simulink model "adcs_v11_log"  (Simulink 7.4)
settings: Solver=ode4  StartTime=0.0  StopTime=80000  FixedStep=s_SIM_STEP_SIZE  RelTol=1e-3
values from neighbouring files (symbols this model uses):
  A = ((T_SIDE + .29)*1e-3)^2    [constants_v13.m]    (also in constants_v15.m; constants_v15_Pow.m; constants_v15_Pow_ss_error.m; constants_v16_integral_kartavya.m)
  Ca_Solar_Drag = 1.4    [constants_v13.m]    (also in constants_v15.m; constants_v15_Pow.m; constants_v15_Pow_ss_error.m; constants_v16_integral_kartavya.m)
  Cd = 2.2    [constants_v13.m]    (also in constants_v15.m; constants_v15_Pow.m; constants_v15_Pow_ss_error.m; constants_v16_integral_kartavya.m)
  check_time = 60000    [constants_v13.m]    (also in constants_v15.m = 10000; constants_v15_Pow.m = 10000; constants_v15_Pow_ss_error.m = 10000; constants_v16_integral_kartavya.m = 10000)
  equinox = datenum('21-Mar-2010 12:0:0')    [constants_v13.m]    (also in constants_v15.m; constants_v15_Pow.m; constants_v15_Pow_ss_error.m; constants_v16_integral_kartavya.m)
  err_SGP = 0    [constants_v16_integral_kartavya.m]    (also in constants_v16_integral_light_sun_sgp_igrf_power_13Dec2011.m)
  I_MAX = 0.5    [constants_v13.m]    (also in constants_v15.m; constants_v15_Pow.m; constants_v15_Pow_ss_error.m; constants_v16_integral_kartavya.m)
  I_TORQUER = 3.6 / 7.31    (= 0.492476060192)    [constants_v13.m]    (also in constants_v15.m; constants_v15_Pow.m; constants_v15_Pow_ss_error.m; constants_v16_integral_kartavya.m)
  Kd = 2* m_INERTIA / (s_numOrbits * T_ORBIT )    [constants_v13.m]    (also in constants_v15.m = m_INERTIA * (2 + delta)* zeta * w; constants_v15_Pow.m = m_INERTIA * (2 + delta)* zeta * w; constants_v15_Pow_ss_error.m = m_INERTIA * (2 + delta)* zeta * w; constants_v16_integral_kartavya.m = m_INERTIA * (2 + delta)* zeta * w)
  Kdetumb = K_det*eye(3)    [constants_v13.m]    (also in constants_v15.m; constants_v15_Pow.m; constants_v15_Pow_ss_error.m; constants_v16_integral_kartavya.m)
  Kp = m_INERTIA / (s_numOrbits * T_ORBIT * zeta)^2    [constants_v13.m]    (also in constants_v15.m = m_INERTIA * (w*w + 2*delta*zeta^2*w^2); constants_v15_Pow.m = m_INERTIA * (w*w + 2*delta*zeta^2*w^2); constants_v15_Pow_ss_error.m = m_INERTIA * (w*w + 2*delta*zeta^2*w^2); constants_v16_integral_kartavya.m = m_INERTIA * (w*w + 2*delta*zeta^2*w^2))
  m_INERTIA = [Ixx Ixy Ixz; Ixy Iyy Iyz; Ixz Iyz Izz]    [constants_v13.m]    (also in constants_v15.m; constants_v15_Pow.m = 1*[Ixx Ixy Ixz; Ixy Iyy Iyz; Ixz Iyz Izz]; constants_v15_Pow_ss_error.m = 1*[Ixx Ixy Ixz; Ixy Iyy Iyz; Ixz Iyz Izz]; constants_v16_integral_kartavya.m)
  mu = 6.673e-11*5.9742e24    (= 398658366000000)    [constants_v13.m]    (also in constants_v15.m; constants_v15_Pow.m; constants_v15_Pow_ss_error.m; constants_v16_integral_kartavya.m)
  N = 40    [constants_v13.m]    (also in constants_v15.m; constants_v15_Pow.m; constants_v15_Pow_ss_error.m; constants_v16_integral_kartavya.m)
  P_momentum_flux_from_the_sun = 4.4e-6    (= 4.4e-06)    [constants_v13.m]    (also in constants_v15.m; constants_v15_Pow.m; constants_v15_Pow_ss_error.m; constants_v16_integral_kartavya.m)
  q_BI0 = euler2qBI(roll0,pitch0,yaw0)    [constants_v13.m]    (also in constants_v15.m; constants_v15_Pow.m; constants_v15_Pow_ss_error.m; constants_v16_integral_kartavya.m)
  s_AU = 159597870610    [constants_v16_integral_kartavya.m]    (also in constants_v16_integral_light_sun_sgp_igrf_power_13Dec2011.m; light_calc.m)
  s_DOY = sime(2)*30 - 30 + sime(3)    [constants_v16_integral_kartavya.m]    (also in constants_v16_integral_light_sun_sgp_igrf_power_13Dec2011.m; precalcs.m)
  s_FRAME_SIZE = 2    [constants_v13.m]    (also in constants_v15.m; constants_v15_Pow.m; constants_v15_Pow_ss_error.m; constants_v16_integral_kartavya.m)
  s_m_MAX = 0.95    [constants_v13.m]    (also in constants_v15.m; constants_v15_Pow.m; constants_v15_Pow_ss_error.m; constants_v16_integral_kartavya.m)
  s_MAG_B = 2.5e-5    (= 2.5e-05)    [constants_v13.m]    (also in constants_v15.m; constants_v15_Pow.m; constants_v15_Pow_ss_error.m; constants_v16_integral_kartavya.m)
  s_MAGMETER_WEIGHT = .9    (= 0.9)    [constants_v13.m]    (also in constants_v15.m; constants_v15_Pow.m; constants_v15_Pow_ss_error.m; constants_v16_integral_kartavya.m)
  s_Rearth = 6378164    [constants_v16_integral_kartavya.m]    (also in constants_v16_integral_light_sun_sgp_igrf_power_13Dec2011.m; light_calc.m)
  s_Rsun = 695500000    [constants_v16_integral_kartavya.m]    (also in constants_v16_integral_light_sun_sgp_igrf_power_13Dec2011.m; light_calc.m)
  s_SEC = sime(4)*3600 + sime(5)*60 + sime(6)    [constants_v16_integral_kartavya.m]    (also in constants_v16_integral_light_sun_sgp_igrf_power_13Dec2011.m; precalcs.m)
  s_SIM_STEP_SIZE = 0.1    [constants_v13.m]    (also in constants_v15.m; constants_v15_Pow.m; constants_v15_Pow_ss_error.m; constants_v16_integral_kartavya.m)
  s_SS_ADC_gain = 5    [constants_v13.m]    (also in constants_v15.m; constants_v15_Pow.m; constants_v15_Pow_ss_error.m; constants_v16_integral_kartavya.m)
  s_SS_ADC_res = 2^12 - 1    (= 4095)    [constants_v13.m]    (also in constants_v15.m; constants_v15_Pow.m; constants_v15_Pow_ss_error.m; constants_v16_integral_kartavya.m)
  s_SS_MAX_ANGLE = 85    [constants_v13.m]    (also in constants_v15.m; constants_v15_Pow.m; constants_v15_Pow_ss_error.m; constants_v16_integral_kartavya.m)
  s_W_SAT = sqrt(mu/R_e^3)    [constants_v13.m]    (also in constants_v15.m; constants_v15_Pow.m; constants_v15_Pow_ss_error.m; constants_v16_integral_kartavya.m)
  s_x_MAGMETER_BIAS = 50e-9    (= 5e-08)    [constants_v13.m]    (also in constants_v15.m; constants_v15_Pow.m; constants_v15_Pow_ss_error.m; constants_v16_integral_kartavya.m)
  s_YEAR = sime(1) + (sime(2)*30 - 30 + sime(3))/365    [constants_v16_integral_kartavya.m]    (also in constants_v16_integral_light_sun_sgp_igrf_power_13Dec2011.m; precalcs.m)
  side = 0.26    [constants_v13.m]    (also in constants_v15.m; constants_v15_Pow.m; constants_v15_Pow_ss_error.m; constants_v16_integral_kartavya.m)
  Snum = 6    [constants_v13.m]    (also in constants_v15.m; constants_v15_Pow.m; constants_v15_Pow_ss_error.m; constants_v16_integral_kartavya.m)
  stperut = 1.00273790935    [constants_v16_integral_kartavya.m]    (also in constants_v16_integral_light_sun_sgp_igrf_power_13Dec2011.m; precalcs.m)
  t_reset = 600    [constants_v16_integral_kartavya.m]    (also in constants_v16_integral_light_sun_sgp_igrf_power_13Dec2011.m; precalcs.m)
  TLE_epoch = datenum('18-Oct-2010 10:30:0')    [constants_v16_integral_kartavya.m]    (also in constants_v16_integral_light_sun_sgp_igrf_power_13Dec2011.m; precalcs.m)
  today = datenum('18-Oct-2010 10:30:0')    [constants_v13.m]    (also in constants_v15.m; constants_v15_Pow.m; constants_v15_Pow_ss_error.m; constants_v16_integral_kartavya.m)
  tol_w = 4e-3    (= 0.004)    [constants_v13.m]    (also in constants_v15.m; constants_v15_Pow.m; constants_v15_Pow_ss_error.m; constants_v16_integral_kartavya.m)
  Ts_display = 6    [constants_v13.m]    (also in constants_v15.m; constants_v15_Pow.m; constants_v15_Pow_ss_error.m; constants_v16_integral_kartavya.m)
  v_COM_to_COP_b = [.2; 1.75; .2]*1e-2    [constants_v13.m]    (also in constants_v15.m; constants_v15_Pow.m; constants_v15_Pow_ss_error.m; constants_v16_integral_kartavya.m)
  v_S1 = [1 0 0]    [constants_v13.m]    (also in constants_v15.m; constants_v15_Pow.m; constants_v15_Pow_ss_error.m; constants_v16_integral_kartavya.m)
  v_S2 = [-1 0 0]    [constants_v13.m]    (also in constants_v15.m; constants_v15_Pow.m; constants_v15_Pow_ss_error.m; constants_v16_integral_kartavya.m)
  v_S3 = [0 1 0]    [constants_v13.m]    (also in constants_v15.m; constants_v15_Pow.m; constants_v15_Pow_ss_error.m; constants_v16_integral_kartavya.m)
  v_S4 = [0 -1 0]    [constants_v13.m]    (also in constants_v15.m; constants_v15_Pow.m; constants_v15_Pow_ss_error.m; constants_v16_integral_kartavya.m)
  v_S5 = [0 0 1]    [constants_v13.m]    (also in constants_v15.m; constants_v15_Pow.m; constants_v15_Pow_ss_error.m; constants_v16_integral_kartavya.m)
  v_S6 = [0 0 -1]    [constants_v13.m]    (also in constants_v15.m; constants_v15_Pow.m; constants_v15_Pow_ss_error.m; constants_v16_integral_kartavya.m)
  v_x_MOUNTING_THETA_ZYX_BODY_TORQUER = [1; 1; 1]* pi/180    [constants_v13.m]    (also in constants_v15.m; constants_v15_Pow.m; constants_v15_Pow_ss_error.m; constants_v16_integral_kartavya.m)
  W_EARTH_ROT = 2*pi/86400    (= 7.27220521664e-05)    [constants_v16_integral_kartavya.m]    (also in constants_v16_integral_light_sun_sgp_igrf_power_13Dec2011.m; precalcs.m)
  wx0 = 2*pi/180    (= 0.0349065850399)    [constants_v13.m]    (also in constants_v15.m = 0.00174532925199; constants_v15_Pow.m = 1.74532925199e-05; constants_v15_Pow_ss_error.m = 2.01533262693e-05; constants_v16_integral_kartavya.m = 0.0174532925199)
  wy0 = 1*pi/180    (= 0.0174532925199)    [constants_v13.m]    (also in constants_v15.m = 0.00174532925199; constants_v15_Pow.m = 1.74532925199e-05; constants_v15_Pow_ss_error.m = 2.01533262693e-05; constants_v16_integral_kartavya.m = 0)
  wz0 = -2*pi/180    (= -0.0349065850399)    [constants_v13.m]    (also in constants_v15.m = 0.00174532925199; constants_v15_Pow.m = 1.74532925199e-05; constants_v15_Pow_ss_error.m = 2.01533262693e-05; constants_v16_integral_kartavya.m = -0.00872664625997)
undefined symbols (not defined in the file or in its folder): Earth, s_omega_MAX, s_YEAR_ONLY, tol_pitch, tol_roll, tol_yaw, v_S10, v_S11, v_S12, v_S7, v_S8, v_S9, v_Si0, WGS84
libraries: commnoisgen2 x15, aerolibutil x7, aerolibtransform2 x5, dspsigops x5, powerlib_extras x3, aerolibgravity2 x2, aerolibatmos2 x1, dspmtrx3 x1, simulink x1
(part 1 of 3)
settings Model: Creator=Jaideep  LastModifiedBy=Jaideep  SimulationMode=rapid-accelerator  ExtModeTrigDuration=100
settings SolverCC: AutoInsertRateTranBlk=on
settings DataIOCC: SaveFinalState=on  SaveOutput=off  SaveState=on  StateSaveName=tmp_raccel_xout
settings OptimizationCC: EfficientMapNaN2IntZero=off
settings HardwareCC: TargetEndianess=LittleEndian  TargetHWDeviceType=MATLAB Host  ProdEqTarget=off
settings RTWCC: SystemTargetFile=raccel.tlc  TemplateMakefile=raccel_default_tmf  RTWVerbose=off  ProcessScript=raccel_make_rtw_hook
settings CodeAppCC: GenerateComments=off  MaxIdLength=128  SimulinkBlockComments=off
settings RaccelTargetCC: TargetFunctionLibrary=ANSI_C  ERTMultiwordTypeDef=System defined  ERTMultiwordLength=256  IsPILTarget=off  ParMdlRefBuildCompliant=off  GeneratePreprocessorConditionals=Disable all  ERTFirstTimeCompliant=off  MultiInstanceERTCode=off  EnableShiftOperators=on  PortableWordSizes=off  ExtModeMexArgs='', 0, 7081  RTWCAPISignals=off  RTWCAPIParams=off

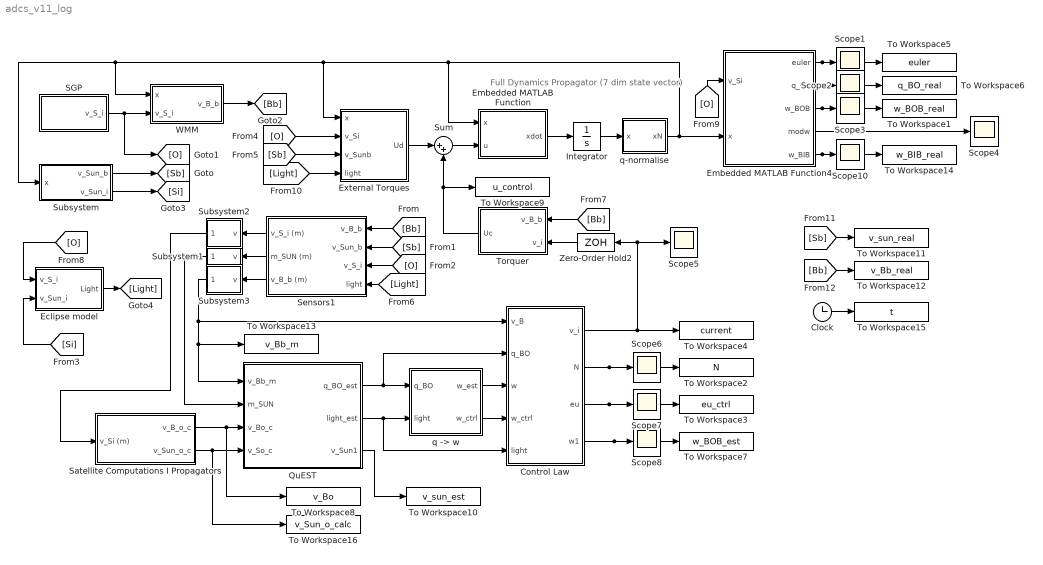
== system adcs_v11_log ==
  note: Full Dynamics Propagator
      |  (7 dim state vector)
  Clock : Clock
      settings: Decimation=10
  Control Law : Subsystem
  Eclipse model : Subsystem
  Embedded MATLAB Function : Stateflow chart
  Embedded MATLAB Function4 : Stateflow chart
  External Torques : Subsystem
  Integrator : Integrator  InitialCondition=[q_BI0; wx0; wy0; wz0]
  QuEST : Stateflow chart
  "SGP " : Subsystem
  Satellite Computations I Propagators : Subsystem
  Scope{1..8,10} (9 alike) : Scope
      Scope1 settings: TimeRange=80000  YMin=-200  YMax=200  SampleInput=on  SampleTime=5
      Scope10 settings: YMin=0.004  YMax=0.0075  SaveName=ScopeData23  SampleInput=on  SampleTime=5
      Scope2 settings: YMin=-10  YMax=10  SaveName=ScopeData7  SampleInput=on  SampleTime=5
      Scope3 settings: YMin=-10  YMax=10  SaveName=ScopeData14  SampleInput=on  SampleTime=5
      Scope4 settings: YMin=0.004  YMax=0.0075  SaveName=ScopeData21  SampleInput=on  SampleTime=5
      Scope5 settings: YMin=-0.045  YMax=0.04  SaveName=ScopeData11  SampleInput=on  SampleTime=5
      Scope6 settings: YMin=-1  YMax=1  SaveName=ScopeData15  SampleInput=on  SampleTime=5
      Scope7 settings: YMin=-10  YMax=10  SaveName=ScopeData16  SampleInput=on  SampleTime=5
      Scope8 settings: YMin=-10  YMax=10  SaveName=ScopeData20  SampleInput=on  SampleTime=5
  Sensors1 : Subsystem
  Subsystem : Subsystem
  Subsystem1 : Subsystem
  Subsystem2 : Subsystem
  Subsystem3 : Subsystem
  Sum : Sum  Inputs=|++  OutDataType=sfix(16)  OutScaling=2^0
  To Workspace1 : ToWorkspace  VariableName=w_BOB_real  SampleTime=Ts_display  SaveFormat=Array
  To Workspace10 : ToWorkspace  VariableName=v_sun_est  SampleTime=Ts_display  SaveFormat=Array
  To Workspace11 : ToWorkspace  VariableName=v_sun_real  SampleTime=Ts_display  SaveFormat=Array
  To Workspace12 : ToWorkspace  VariableName=v_Bb_real  SampleTime=Ts_display  SaveFormat=Array
  To Workspace13 : ToWorkspace  VariableName=v_Bb_m  SampleTime=Ts_display  SaveFormat=Array
  To Workspace14 : ToWorkspace  VariableName=w_BIB_real  SampleTime=Ts_display  SaveFormat=Array
  To Workspace15 : ToWorkspace  VariableName=t  SampleTime=Ts_display  SaveFormat=Array
  To Workspace16 : ToWorkspace  VariableName=v_Sun_o_calc  SampleTime=Ts_display  SaveFormat=Array
  To Workspace2 : ToWorkspace  VariableName=N  SampleTime=Ts_display  SaveFormat=Array
  To Workspace3 : ToWorkspace  VariableName=eu_ctrl  SampleTime=Ts_display  SaveFormat=Array
  To Workspace4 : ToWorkspace  VariableName=current  SampleTime=Ts_display  SaveFormat=Array
  To Workspace5 : ToWorkspace  VariableName=euler  SampleTime=Ts_display  SaveFormat=Array
  To Workspace6 : ToWorkspace  VariableName=q_BO_real  SampleTime=Ts_display  SaveFormat=Array
  To Workspace7 : ToWorkspace  VariableName=w_BOB_est  SampleTime=Ts_display  SaveFormat=Array
  To Workspace8 : ToWorkspace  VariableName=v_Bo  SampleTime=Ts_display  SaveFormat=Array
  To Workspace9 : ToWorkspace  VariableName=u_control  SampleTime=Ts_display  SaveFormat=Array
  Torquer : Subsystem
  WMM : Subsystem
  Zero-Order Hold2 : ZeroOrderHold  SampleTime=s_FRAME_SIZE
  "q -> w" : Subsystem
  q-normalise : Stateflow chart
  wires:
  Embedded MATLAB Function/1(xdot) -> Integrator/1
  Integrator/1 -> q-normalise/1(x)
  "SGP "/1(v_S_i) -> WMM/2(v_S_i), [O]
  q-normalise/1(xN) -> Subsystem/1(x), WMM/1(x), External Torques/1(x), Embedded MATLAB Function/1(x), Embedded MATLAB Function4/2(x)
  Sum/1 -> Embedded MATLAB Function/2(u)
  WMM/1(v_B_b) -> [Bb]
  Subsystem/1(v_Sun_b) -> [Sb]
  [Bb] -> Sensors1/1(v_B_b)
  [Sb] -> Sensors1/2(v_Sun_b)
  Subsystem/2(v_Sun_i) -> [Si]
  [O] -> External Torques/2(v_Si)
  [Sb] -> External Torques/3(v_Sunb)
  [Bb] -> Torquer/1(v_B_b)
  [O] -> Sensors1/3(v_S_i)
  [Light] -> Sensors1/4(light)
  Sensors1/1(v_S_i (m)) -> Subsystem2/1(v)
  [Si] -> Eclipse model/2(v_Sun_i)
  [O] -> Eclipse model/1(v_S_i)
  Sensors1/2(m_SUN (m)) -> Subsystem1/1(v)
  Sensors1/3(v_B_b (m)) -> Subsystem3/1(v)
  Zero-Order Hold2/1 -> Torquer/2(v_i)
  External Torques/1(Ud) -> Sum/1
  Torquer/1(Uc) -> Sum/2, To Workspace9/1
  Subsystem2/1(v(H)) -> Satellite Computations I Propagators/1(v_Si (m))
  Subsystem1/1(v(H)) -> QuEST/2(m_SUN)
  Subsystem3/1(v(H)) -> Control Law/1(v_B), QuEST/1(v_Bb_m), To Workspace13/1
  Satellite Computations I Propagators/1(v_B_o_c) -> QuEST/3(v_Bo_c), To Workspace8/1
  Satellite Computations I Propagators/2(v_Sun_o_c) -> QuEST/4(v_So_c), To Workspace16/1
  QuEST/1(q_BO_est) -> Control Law/2(q_BO), "q -> w"/1(q_BO)
  QuEST/2(light_est) -> "q -> w"/2(light), Control Law/5(light)
  Control Law/1(v_i) -> To Workspace4/1, Zero-Order Hold2/1, Scope5/1
  Embedded MATLAB Function4/2(q_BO) -> Scope2/1, To Workspace6/1
  Embedded MATLAB Function4/1(euler) -> Scope1/1, To Workspace5/1
  [O] -> Embedded MATLAB Function4/1(v_Si)
  Control Law/2(N) -> Scope6/1, To Workspace2/1
  Eclipse model/1(Light) -> [Light]
  Control Law/3(eu) -> Scope7/1, To Workspace3/1
  Embedded MATLAB Function4/3(w_BOB) -> Scope3/1, To Workspace1/1
  Embedded MATLAB Function4/4(modw) -> Scope4/1
  Control Law/4(w1) -> Scope8/1, To Workspace7/1
  "q -> w"/1(w_est) -> Control Law/3(w)
  [Light] -> External Torques/4(light)
  "q -> w"/2(w_ctrl) -> Control Law/4(w_ctrl)
  QuEST/3(v_Sun1) -> To Workspace10/1
  [Sb] -> To Workspace11/1
  [Bb] -> To Workspace12/1
  Embedded MATLAB Function4/5(w_BIB) -> Scope10/1, To Workspace14/1
  Clock/1 -> To Workspace15/1

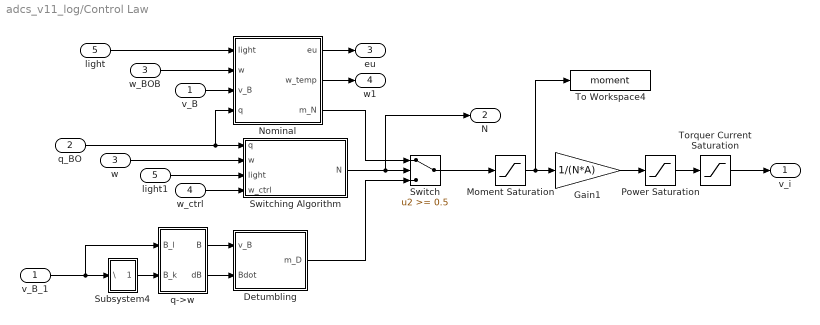
== system adcs_v11_log/Control Law ==
  v_B : Inport  OutDataType=sfix(16)  OutScaling=2^0
  q_BO : Inport  Port=2  OutDataType=sfix(16)  OutScaling=2^0
  w : Inport  Port=3  OutDataType=sfix(16)  OutScaling=2^0
  w_ctrl : Inport  Port=4  OutDataType=sfix(16)  OutScaling=2^0
  light : Inport  Port=5  OutDataType=sfix(16)  OutScaling=2^0
  Detumbling : Stateflow chart
  Gain1 : Gain  Gain=1/(N*A)  ParameterDataType=sfix(16)  ParameterScaling=2^0  OutDataType=sfix(16)  OutScaling=2^0
  Moment Saturation : Saturate  UpperLimit=s_m_MAX  LowerLimit=-s_m_MAX  OutDataType=sfix(16)  OutScaling=2^0
  Nominal : Stateflow chart
  Power Saturation : Saturate  UpperLimit=I_MAX  LowerLimit=-I_MAX  OutDataType=sfix(16)  OutScaling=2^0
  Subsystem4 : Subsystem
  Switch : Switch  Threshold=0.5  OutDataType=sfix(16)  OutScaling=2^0
  Switching Algorithm : Subsystem
  To Workspace4 : ToWorkspace  VariableName=moment  SampleTime=Ts_display  SaveFormat=Array
  Torquer Current Saturation : Saturate  UpperLimit=I_TORQUER  LowerLimit=-I_TORQUER  OutDataType=sfix(16)  OutScaling=2^0
  light1 : InportShadow  Port=5  OutDataType=sfix(16)  OutScaling=2^0  LatchByCopyingInsideSignal=off
  q->w : Stateflow chart
  v_B_1 : InportShadow  Port=1  OutDataType=sfix(16)  OutScaling=2^0  LatchByCopyingInsideSignal=off
  w_BOB : InportShadow  Port=3  OutDataType=sfix(16)  OutScaling=2^0  LatchByCopyingInsideSignal=off
  v_i : Outport  OutDataType=sfix(16)  OutScaling=2^0
  N : Outport  Port=2  OutDataType=sfix(16)  OutScaling=2^0
  eu : Outport  Port=3  OutDataType=sfix(16)  OutScaling=2^0
  w1 : Outport  Port=4  OutDataType=sfix(16)  OutScaling=2^0
  wires:
  q->w/1(B) -> Detumbling/1(v_B)
  Subsystem4/1(=>\) -> q->w/2(B_k)
  q_BO/1 -> Nominal/4(q), Switching Algorithm/1(q)
  light/1 -> Nominal/1(light)
  Gain1/1 -> Power Saturation/1
  Torquer Current Saturation/1 -> v_i/1
  Moment Saturation/1 -> Gain1/1, To Workspace4/1
  Power Saturation/1 -> Torquer Current Saturation/1
  Switch/1 -> Moment Saturation/1
  Detumbling/1(m_D) -> Switch/3
  Switching Algorithm/1(N) -> N/1, Switch/2
  Nominal/3(m_N) -> Switch/1
  w/1 -> Switching Algorithm/2(w)
  v_B_1/1 -> q->w/1(B_l), Subsystem4/1(\)
  q->w/2(dB) -> Detumbling/2(Bdot)
  v_B/1 -> Nominal/3(v_B)
  light1/1 -> Switching Algorithm/3(light)
  w_BOB/1 -> Nominal/2(w)
  Nominal/1(eu) -> eu/1
  Nominal/2(w_temp) -> w1/1
  w_ctrl/1 -> Switching Algorithm/4(w_ctrl)

== system adcs_v11_log/Eclipse model ==
  v_S_i : Inport  OutDataType=sfix(16)  OutScaling=2^0
  v_Sun_i : Inport  Port=2  OutDataType=sfix(16)  OutScaling=2^0
  Constant : Constant  Value=s_AU  OutDataType=sfix(16)  OutScaling=2^0
  Constant1 : Constant  Value=s_Rearth  OutDataType=sfix(16)  OutScaling=2^0
  Constant2 : Constant  Value=s_Rsun  OutDataType=sfix(16)  OutScaling=2^0
  Eclipse Model : Stateflow chart
  Scope{1..4} (4 alike) : Scope
      Scope1 settings: TimeRange=80000  YMin=-6.5  YMax=1  SaveName=ScopeData3  SampleInput=on  SampleTime=5
      Scope2 settings: TimeRange=80000  YMin=-6.5  YMax=1  SaveName=ScopeData4  SampleInput=on  SampleTime=5
      Scope3 settings: TimeRange=80000  YMin=-6.5  YMax=1  SaveName=ScopeData5  SampleInput=on  SampleTime=5
      Scope4 settings: TimeRange=80000  YMin=-6.5  YMax=1  SaveName=ScopeData6  SampleInput=on  SampleTime=5
  Light : Outport  OutDataType=sfix(16)  OutScaling=2^0
  wires:
  Constant/1 -> Eclipse Model/1(s_AU)
  Constant1/1 -> Eclipse Model/2(s_Rearth)
  Constant2/1 -> Eclipse Model/3(s_Rsun)
  Eclipse Model/1(flag) -> Light/1
  v_S_i/1 -> Eclipse Model/4(v_S_i)
  v_Sun_i/1 -> Eclipse Model/5(v_Sun_i)
  Eclipse Model/2(alpha) -> Scope1/1
  Eclipse Model/3(beta) -> Scope2/1
  Eclipse Model/4(parameter_umbra) -> Scope3/1
  Eclipse Model/5(parameter_penumbra) -> Scope4/1

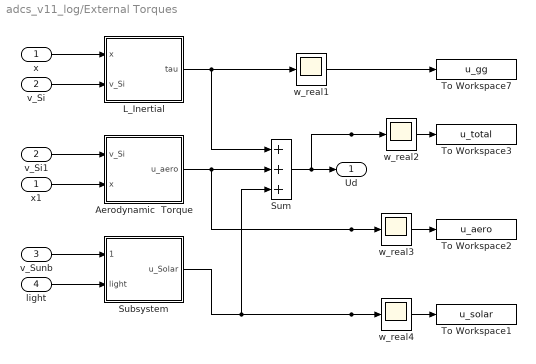
== system adcs_v11_log/External Torques ==
  x : Inport  OutDataType=sfix(16)  OutScaling=2^0
  v_Si : Inport  Port=2  OutDataType=sfix(16)  OutScaling=2^0
  v_Sunb : Inport  Port=3  OutDataType=sfix(16)  OutScaling=2^0
  light : Inport  Port=4  OutDataType=sfix(16)  OutScaling=2^0
  Aerodynamic  Torque : Subsystem
  L_Inertial : Stateflow chart
  Subsystem : Subsystem
  Sum : Sum  Inputs=+++  OutDataType=fixdt(1, 16)  OutScaling=2^0
  To Workspace1 : ToWorkspace  VariableName=u_solar  SampleTime=Ts_display  SaveFormat=Array
  To Workspace2 : ToWorkspace  VariableName=u_aero  SampleTime=Ts_display  SaveFormat=Array
  To Workspace3 : ToWorkspace  VariableName=u_total  SampleTime=Ts_display  SaveFormat=Array
  To Workspace7 : ToWorkspace  VariableName=u_gg  SampleTime=Ts_display  SaveFormat=Array
  v_Si1 : InportShadow  Port=2  OutDataType=sfix(16)  OutScaling=2^0  LatchByCopyingInsideSignal=off
  w_real{1..4} (4 alike) : Scope
      w_real1 settings: YMin=-3e-009  YMax=1.1e-008  SaveName=ScopeData18  SampleInput=on  SampleTime=5
      w_real2 settings: YMin=-7e-009  YMax=1e-008  SaveName=ScopeData17  SampleInput=on  SampleTime=5
      w_real3 settings: YMin=-8e-010  YMax=1.4e-009  SaveName=ScopeData19  SampleInput=on  SampleTime=5
      w_real4 settings: YMin=-6e-009  YMax=1e-008  SaveName=ScopeData22  SampleInput=on  SampleTime=5
  x1 : InportShadow  Port=1  OutDataType=sfix(16)  OutScaling=2^0  LatchByCopyingInsideSignal=off
  Ud : Outport  OutDataType=sfix(16)  OutScaling=2^0
  wires:
  x/1 -> L_Inertial/1(x)
  v_Si/1 -> L_Inertial/2(v_Si)
  L_Inertial/1(tau) -> Sum/1, w_real1/1, To Workspace7/1
  Aerodynamic  Torque/1(u_aero) -> Sum/2, w_real3/1, To Workspace2/1
  x1/1 -> Aerodynamic  Torque/2(x)
  v_Si1/1 -> Aerodynamic  Torque/1(v_Si)
  Sum/1 -> Ud/1, w_real2/1, To Workspace3/1
  v_Sunb/1 -> Subsystem/1(v_Sun_b)
  Subsystem/1(u_Solar) -> Sum/3, w_real4/1, To Workspace1/1
  light/1 -> Subsystem/2(light)

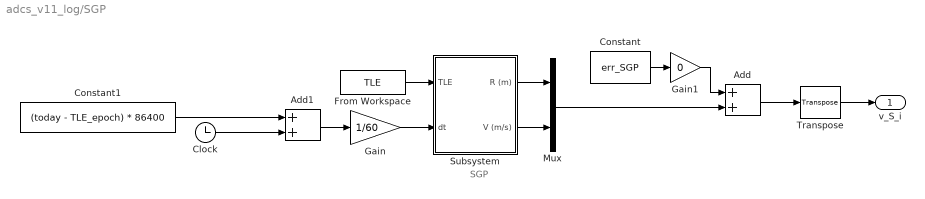
== system adcs_v11_log/SGP  ==
  note: SGP
  Add : Sum  OutDataType=sfix(16)  OutScaling=2^-10
  Add1 : Sum  OutDataType=sfix(16)  OutScaling=2^-10
  Clock : Clock
      settings: Decimation=10
  Constant : Constant  Value=err_SGP  VectorParams1D=off  OutDataType=sfix(16)  OutScaling=2^0
  Constant1 : Constant  Value=(today - TLE_epoch) * 86400  VectorParams1D=off  OutDataType=sfix(16)  OutScaling=2^0
  From Workspace : FromWorkspace  VariableName=TLE  SampleTime=0
  Gain : Gain  Gain=1/60  ParameterDataType=sfix(16)  ParameterScaling=2^0  OutDataType=sfix(16)  OutScaling=2^0
  Gain1 : Gain  Gain=0  ParameterDataType=sfix(16)  ParameterScaling=2^0  OutDataType=sfix(16)  OutScaling=2^0
  Mux : Mux  Inputs=2
  Subsystem : Subsystem
  Transpose : dspmtrx3/Transpose  SystemSampleTime=-1  Hermitian=off  overflowFlag=off
  v_S_i : Outport  OutDataType=sfix(16)  OutScaling=2^0
  wires:
  Transpose/1 -> v_S_i/1
  Gain1/1 -> Add/1
  Add1/1 -> Gain/1
  Clock/1 -> Add1/2
  Constant1/1 -> Add1/1
  Add/1 -> Transpose/1
  Constant/1 -> Gain1/1
  Gain/1 -> Subsystem/2(dt)
  Mux/1 -> Add/2
  Subsystem/2(V (m/s)) -> Mux/2
  Subsystem/1(R (m)) -> Mux/1
  From Workspace/1 -> Subsystem/1(TLE)

== system adcs_v11_log/Satellite Computations I Propagators ==
  v_Si (m) : Inport  OutDataType=sfix(16)  OutScaling=2^0
  Orbit propagator model : Subsystem
  Subsystem : Subsystem
  WMM : Subsystem
  m_TOI_NEW : Stateflow chart
  m_TOI_NEW1 : Stateflow chart
  v_B_o_c : Outport  OutDataType=sfix(16)  OutScaling=2^0
  v_Sun_o_c : Outport  Port=2  OutDataType=sfix(16)  OutScaling=2^0
  wires:
  Orbit propagator model/1(v_S_i (m)) -> m_TOI_NEW1/2(ECI), m_TOI_NEW/1(ECI), WMM/1(v_Si)
  WMM/1(v_Bi_c) -> m_TOI_NEW/2(v_I)
  v_Si (m)/1 -> Orbit propagator model/1(v_State_i measured by GPS)
  m_TOI_NEW1/1(v_O) -> v_Sun_o_c/1
  m_TOI_NEW/1(v_O) -> v_B_o_c/1
  Subsystem/1(v_Sun_I_c) -> m_TOI_NEW1/1(v_I)

== system adcs_v11_log/Sensors1 ==
  note: 'm' stands for measured
  v_B_b : Inport  OutDataType=sfix(16)  OutScaling=2^0
  v_Sun_b : Inport  Port=2  OutDataType=sfix(16)  OutScaling=2^0
  v_S_i : Inport  Port=3  OutDataType=sfix(16)  OutScaling=2^0
  light : Inport  Port=4  OutDataType=sfix(16)  OutScaling=2^0
  GPS : Subsystem
  Magnetometer simple : Subsystem
  Sun Sensors : Subsystem
  v_S_i (m) : Outport  OutDataType=sfix(16)  OutScaling=2^0
  m_SUN (m) : Outport  Port=2  OutDataType=sfix(16)  OutScaling=2^0
  v_B_b (m) : Outport  Port=3  OutDataType=sfix(16)  OutScaling=2^0
  wires:
  light/1 -> Sun Sensors/2(Light)
  GPS/1(v_S_i (m)) -> v_S_i (m)/1
  v_S_i/1 -> GPS/1(v_S_i)
  Magnetometer simple/1(v_B_b(m)) -> v_B_b (m)/1
  v_B_b/1 -> Magnetometer simple/1(v_B_b)
  v_Sun_b/1 -> Sun Sensors/1(v_Sun_b)
  Sun Sensors/1(m_SUN) -> m_SUN (m)/1

== system adcs_v11_log/Subsystem ==
  x : Inport  OutDataType=sfix(16)  OutScaling=2^0
  Clock : Clock
      settings: Decimation=10
  Constant : Constant  Value=today-equinox  OutDataType=sfix(16)  OutScaling=2^0
  Sun Vector Propagator : Stateflow chart
  To Workspace8 : ToWorkspace  VariableName=v_Sun_i  SampleTime=Ts_display  SaveFormat=Array
  f: I->B : Stateflow chart
  v_Sun_b : Outport  OutDataType=sfix(16)  OutScaling=2^0
  v_Sun_i : Outport  Port=2  OutDataType=sfix(16)  OutScaling=2^0
  wires:
  x/1 -> f: I->B/1(x)
  f: I->B/1(v_B) -> v_Sun_b/1
  Sun Vector Propagator/1(v_Sun_i) -> f: I->B/2(v_I), v_Sun_i/1, To Workspace8/1
  Clock/1 -> Sun Vector Propagator/2(t)
  Constant/1 -> Sun Vector Propagator/1(today)

== system adcs_v11_log/Subsystem1 ==
  v : Inport
  Pulse Generator : DiscretePulseGenerator  PulseType=Time based  Amplitude=1  Period=s_FRAME_SIZE  PulseWidth=50  PhaseDelay=0  SampleTime=1
  Sample and Hold : dspsigops/Sample and Hold  SystemSampleTime=-1  trig=Rising edge  initCond=m_SUN0  latchinput=off
  v(H) : Outport
  wires:
  Sample and Hold/1 -> v(H)/1
  v/1 -> Sample and Hold/1
  Pulse Generator/1 -> Sample and Hold/Trigger

== system adcs_v11_log/Subsystem2 ==
  v : Inport
  Pulse Generator : DiscretePulseGenerator  PulseType=Time based  Amplitude=1  Period=s_FRAME_SIZE  PulseWidth=50  PhaseDelay=0  SampleTime=1
  Sample and Hold : dspsigops/Sample and Hold  SystemSampleTime=-1  trig=Rising edge  initCond=v_Si0  latchinput=off
  v(H) : Outport
  wires:
  Pulse Generator/1 -> Sample and Hold/Trigger
  v/1 -> Sample and Hold/1
  Sample and Hold/1 -> v(H)/1

== system adcs_v11_log/Subsystem3 ==
  v : Inport
  Pulse Generator : DiscretePulseGenerator  PulseType=Time based  Amplitude=1  Period=s_FRAME_SIZE  PulseWidth=50  PhaseDelay=0  SampleTime=1
  Sample and Hold : dspsigops/Sample and Hold  SystemSampleTime=-1  trig=Rising edge  initCond=v_Bb0  latchinput=off
  v(H) : Outport
  wires:
  Sample and Hold/1 -> v(H)/1
  v/1 -> Sample and Hold/1
  Pulse Generator/1 -> Sample and Hold/Trigger

== system adcs_v11_log/Torquer ==
  v_B_b : Inport  OutDataType=sfix(16)  OutScaling=2^0
  v_i : Inport  Port=2  OutDataType=sfix(16)  OutScaling=2^0
  3x3 Cross Product : aerolibutil/3x3 Cross Product  SystemSampleTime=-1
  Constant : Constant  Value=v_x_MOUNTING_THETA_ZYX_BODY_TORQUER  OutDataType=sfix(16)  OutScaling=2^0
  Embedded MATLAB Function4 : Stateflow chart
  Gain : Gain  Gain=0  ParameterDataType=sfix(16)  ParameterScaling=2^0  OutDataType=sfix(16)  OutScaling=2^0
  Gain2 : Gain  Gain=N*A  ParameterDataType=sfix(16)  ParameterScaling=2^0  OutDataType=sfix(16)  OutScaling=2^0
  PWM : Quantizer  QuantizationInterval=s_PWM_RES
  Product : Product  Multiplication=Matrix(*)  OutDataType=sfix(16)  OutScaling=2^0  RndMeth=Zero
  Uc : Outport  OutDataType=sfix(16)  OutScaling=2^0
  wires:
  PWM/1 -> Gain2/1
  v_B_b/1 -> 3x3 Cross Product/2
  3x3 Cross Product/1 -> Uc/1
  v_i/1 -> PWM/1
  Embedded MATLAB Function4/1(DCM) -> Product/1
  Gain2/1 -> Product/2
  Product/1 -> 3x3 Cross Product/1
  Constant/1 -> Gain/1
  Gain/1 -> Embedded MATLAB Function4/1(euler)

== system adcs_v11_log/WMM ==
  x : Inport  OutDataType=sfix(16)  OutScaling=2^0
  v_S_i : Inport  Port=2  OutDataType=sfix(16)  OutScaling=2^0
  L_Inertial : Stateflow chart
  To Workspace8 : ToWorkspace  VariableName=v_Bi  SampleTime=Ts_display  SaveFormat=Array
  state vector to v_Bi : Subsystem
  v_B_b : Outport  OutDataType=sfix(16)  OutScaling=2^0
  wires:
  L_Inertial/1(v_B) -> v_B_b/1
  x/1 -> L_Inertial/1(x)
  v_S_i/1 -> state vector to v_Bi/1(v_S_i)
  state vector to v_Bi/1(v_B_I) -> L_Inertial/2(v_I), To Workspace8/1

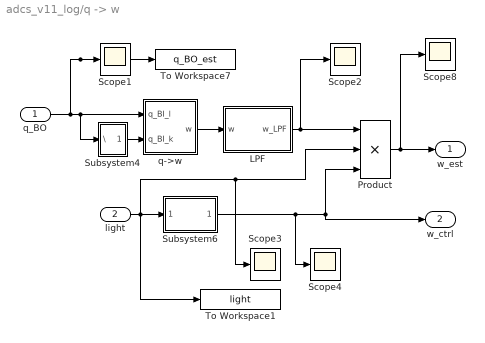
== system adcs_v11_log/q -> w ==
  q_BO : Inport
  light : Inport  Port=2
  LPF : Subsystem
  Product : Product  Inputs=3  OutDataType=fixdt(1, 16)  OutScaling=2^0  RndMeth=Zero
  Scope{1..4,8} (5 alike) : Scope
      Scope1 settings: YMin=-0.8  YMax=0.9  SaveName=ScopeData9  SampleInput=on  SampleTime=5
      Scope2 settings: YMin=-4.5e-012  YMax=2.5e-012  SaveName=ScopeData8  SampleInput=on  SampleTime=5
      Scope3 settings: YMin=-4.5e-012  YMax=2.5e-012  SaveName=ScopeData24  SampleInput=on  SampleTime=5
      Scope4 settings: YMin=-1  YMax=1  SaveName=ScopeData25  SampleInput=on  SampleTime=5
      Scope8 settings: YMin=-1  YMax=1  SaveName=ScopeData13  SampleInput=on  SampleTime=5
  Subsystem4 : Subsystem
  Subsystem6 : Subsystem
  To Workspace1 : ToWorkspace  VariableName=light  SampleTime=Ts_display  SaveFormat=Array
  To Workspace7 : ToWorkspace  VariableName=q_BO_est  SampleTime=Ts_display  SaveFormat=Array
  q->w : Stateflow chart
  w_est : Outport
  w_ctrl : Outport  Port=2
  wires:
  q->w/1(w) -> LPF/1("w ")
  LPF/1(w_LPF) -> Product/1, Scope2/1
  Subsystem4/1(=>\) -> q->w/2(q_BI_k)
  Product/1 -> w_est/1, Scope8/1
  light/1 -> Product/2, Scope3/1, Subsystem6/1(light), To Workspace1/1
  q_BO/1 -> q->w/1(q_BI_l), Subsystem4/1(\), Scope1/1, To Workspace7/1
  Subsystem6/1(w-ctrl) -> Product/3, w_ctrl/1, Scope4/1

== system adcs_v11_log/Control Law/Subsystem4 ==
  \ : Inport
  Constant : Constant  Value=s_FRAME_SIZE  OutDataType=fixdt(1, 16)  OutScaling=2^0
  Variable Time Delay : VariableTransportDelay
  =>\ : Outport
  wires:
  Variable Time Delay/1 -> =>\/1
  \/1 -> Variable Time Delay/1
  Constant/1 -> Variable Time Delay/2

== system adcs_v11_log/Control Law/Switching Algorithm ==
  note: remov the t=0 checking
      | code, not necessary
  q : Inport  OutDataType=sfix(16)  OutScaling=2^0
  w : Inport  Port=2  OutDataType=sfix(16)  OutScaling=2^0
  light : Inport  Port=3  OutDataType=sfix(16)  OutScaling=2^0
  w_ctrl : Inport  Port=4  OutDataType=sfix(16)  OutScaling=2^0
  Clock : Clock
      settings: Decimation=10
  Unit Delay : UnitDelay  SampleTime=-1
  gate pulse : Stateflow chart
  N : Outport  OutDataType=sfix(16)  OutScaling=2^0
  wires:
  w/1 -> gate pulse/1(w)
  Clock/1 -> gate pulse/3(t)
  gate pulse/2(time1) -> Unit Delay/1
  Unit Delay/1 -> gate pulse/6(time2)
  q/1 -> gate pulse/2(q)
  gate pulse/1(N) -> N/1
  light/1 -> gate pulse/4(light_flag)
  w_ctrl/1 -> gate pulse/5(w_ctrl)

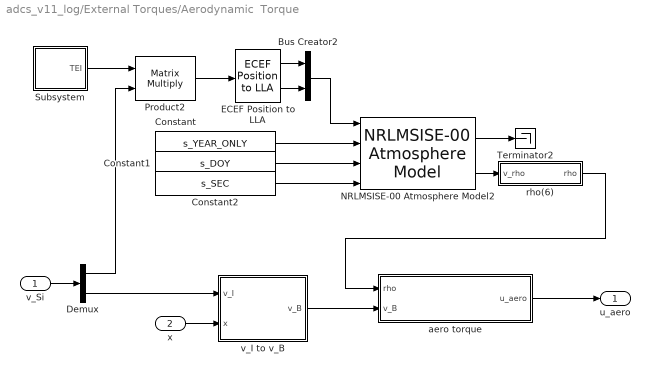
== system adcs_v11_log/External Torques/Aerodynamic  Torque ==
  v_Si : Inport
  x : Inport  Port=2
  Bus Creator2 : BusCreator  Inputs=2
  Constant : Constant  Value=s_YEAR_ONLY  OutDataType=fixdt(1, 16)  OutScaling=2^0
  Constant1 : Constant  Value=s_DOY  OutDataType=fixdt(1, 16)  OutScaling=2^0
  Constant2 : Constant  Value=s_SEC  OutDataType=fixdt(1, 16)  OutScaling=2^0
  Demux : Demux  Outputs=2
  ECEF Position to LLA : aerolibtransform2/ECEF Position to LLA  SystemSampleTime=-1  units=Metric (MKS)  ptype=Earth (WGS84)  F=1/298.257223563  R=6378137
  NRLMSISE-00 Atmosphere Model2 : aerolibatmos2/NRLMSISE-00 Atmosphere Model  SystemSampleTime=-1  units=Metric (MKS)  lst_input=off  flux_ap_input=off  flags_input=Internal  flags=ones(1,23)  oxygen_in=off  action=Warning
  Product2 : Product  Multiplication=Matrix(*)  OutDataType=sfix(16)  OutScaling=2^0  RndMeth=Zero
  Subsystem : Subsystem
  Terminator2 : Terminator
  aero torque : Stateflow chart
  rho(6) : Stateflow chart
  v_I to v_B : Stateflow chart
  u_aero : Outport  OutDataType=sfix(16)  OutScaling=2^0
  wires:
  v_I to v_B/1(v_B) -> aero torque/2(v_B)
  Subsystem/1(TEI) -> Product2/1
  Product2/1 -> ECEF Position to LLA/1
  ECEF Position to LLA/1 -> Bus Creator2/1
  ECEF Position to LLA/2 -> Bus Creator2/2
  Bus Creator2/1 -> NRLMSISE-00 Atmosphere Model2/1
  NRLMSISE-00 Atmosphere Model2/1 -> Terminator2/1
  NRLMSISE-00 Atmosphere Model2/2 -> rho(6)/1(v_rho)
  v_Si/1 -> Demux/1
  Demux/2 -> v_I to v_B/1(v_I)
  x/1 -> v_I to v_B/2(x)
  Demux/1 -> Product2/2
  rho(6)/1(rho) -> aero torque/1(rho)
  Constant/1 -> NRLMSISE-00 Atmosphere Model2/2
  Constant1/1 -> NRLMSISE-00 Atmosphere Model2/3
  Constant2/1 -> NRLMSISE-00 Atmosphere Model2/4
  aero torque/1(u_aero) -> u_aero/1

== system adcs_v11_log/External Torques/Subsystem ==
  v_Sun_b : Inport  OutDataType=sfix(16)  OutScaling=2^0
  light : Inport  Port=2  OutDataType=sfix(16)  OutScaling=2^0
  Solar_drag : Stateflow chart
  Vector from CoM to CoP_in Body frame (yet to be finalized)2 : Constant  Value=v_COM_to_COP_b  VectorParams1D=off  OutDataType=sfix(16)  OutScaling=2^0
  _ : aerolibutil/3x3 Cross Product  SystemSampleTime=-1
  u_Solar : Outport  OutDataType=sfix(16)  OutScaling=2^0
  wires:
  _/1 -> u_Solar/1
  v_Sun_b/1 -> Solar_drag/1(v_Sun_b)
  light/1 -> Solar_drag/2(light)
  Solar_drag/1(solar_drag) -> _/2
  Vector from CoM to CoP_in Body frame (yet to be finalized)2/1 -> _/1

== system adcs_v11_log/SGP /Subsystem ==
  TLE : Inport
  dt : Inport  Port=2
  Embedded MATLAB Function1 : Stateflow chart
  Embedded MATLAB Function2 : Stateflow chart
  R (m) : Outport
  V (m/s) : Outport  Port=2
  wires:
  TLE/1 -> Embedded MATLAB Function1/1(TLE)
  Embedded MATLAB Function2/2(dR) -> V (m/s)/1
  dt/1 -> Embedded MATLAB Function2/2(dT)
  Embedded MATLAB Function2/1(R) -> R (m)/1
  Embedded MATLAB Function1/1(modTLE) -> Embedded MATLAB Function2/1(modTLE)

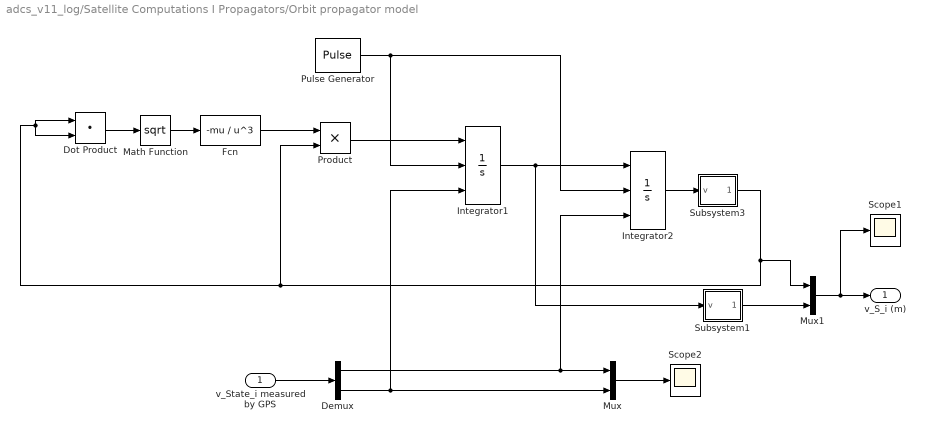
== system adcs_v11_log/Satellite Computations I Propagators/Orbit propagator model ==
  v_State_i measured by GPS : Inport
  Demux : Demux  Outputs=2
  Dot Product : DotProduct  OutDataType=sfix(16)  OutScaling=2^-10  InputSameDT=on  OutDataTypeStr=Inherit: Inherit via internal rule
  Fcn : Fcn  Expr=-mu / u^3
  Integrator1 : Integrator  ExternalReset=rising  InitialConditionSource=external
  Integrator2 : Integrator  ExternalReset=rising  InitialConditionSource=external
  Math Function : Math  Operator=sqrt  OutDataType=sfix(16)  OutScaling=2^0  SaturateOnIntegerOverflow=on
  Mux : Mux  Inputs=2
  Mux1 : Mux  Inputs=2
  Product : Product  OutDataType=sfix(16)  OutScaling=2^0  RndMeth=Zero
  Pulse Generator : DiscretePulseGenerator  PulseType=Time based  Amplitude=1  Period=t_reset  PulseWidth=5  PhaseDelay=0  SampleTime=1
  Scope1 : Scope
      settings: SaveName=ScopeData26  SampleInput=on  SampleTime=5
  Scope2 : Scope
      settings: SaveName=ScopeData27  SampleInput=on  SampleTime=5
  Subsystem1 : Subsystem
  Subsystem3 : Subsystem
  v_S_i (m) : Outport  OutDataType=sfix(16)  OutScaling=2^0
  wires:
  Pulse Generator/1 -> Integrator1/2, Integrator2/2
  Mux/1 -> Scope2/1
  Math Function/1 -> Fcn/1
  Dot Product/1 -> Math Function/1
  v_State_i measured by GPS/1 -> Demux/1
  Demux/1 -> Mux/1, Integrator2/3
  Demux/2 -> Mux/2, Integrator1/3
  Integrator2/1 -> Subsystem3/1(v)
  Integrator1/1 -> Integrator2/1, Subsystem1/1(v)
  Product/1 -> Integrator1/1
  Fcn/1 -> Product/1
  Mux1/1 -> v_S_i (m)/1, Scope1/1
  Subsystem3/1(v(H)) -> Mux1/1, Dot Product/2, Dot Product/1, Product/2
  Subsystem1/1(v(H)) -> Mux1/2

== system adcs_v11_log/Satellite Computations I Propagators/Subsystem ==
  Clock : Clock
      settings: Decimation=10
  Constant : Constant  Value=today-equinox  OutDataType=sfix(16)  OutScaling=2^0
  Embedded MATLAB Function : Stateflow chart
  v_Sun_I_c : Outport  OutDataType=sfix(16)  OutScaling=2^0
  wires:
  Embedded MATLAB Function/1(v_Sun_i) -> v_Sun_I_c/1
  Clock/1 -> Embedded MATLAB Function/2(t)
  Constant/1 -> Embedded MATLAB Function/1(today)

== system adcs_v11_log/Satellite Computations I Propagators/WMM ==
  v_Si : Inport  OutDataType=sfix(16)  OutScaling=2^0
  Demux : Demux  Outputs=2
  Invert  3x3 Matrix : aerolibutil/Invert  3x3 Matrix  SystemSampleTime=-1
  Magnetic field v_Be : Subsystem
  Subsystem : Subsystem
  Terminator : Terminator
  v_Bi : Product  Multiplication=Matrix(*)  OutDataType=sfix(16)  OutScaling=2^0  RndMeth=Zero
  v_Vi1 : Product  Multiplication=Matrix(*)  OutDataType=sfix(16)  OutScaling=2^0  RndMeth=Zero
  v_Bi_c : Outport  OutDataType=sfix(16)  OutScaling=2^0
  wires:
  v_Bi/1 -> v_Bi_c/1
  Demux/1 -> v_Vi1/2
  v_Si/1 -> Demux/1
  Demux/2 -> Terminator/1
  v_Vi1/1 -> Magnetic field v_Be/1(XYZ-ECEF)
  Subsystem/1(TEI) -> v_Vi1/1, Invert  3x3 Matrix/1
  Magnetic field v_Be/1("v_B_e (T) ") -> v_Bi/2
  Invert  3x3 Matrix/1 -> v_Bi/1

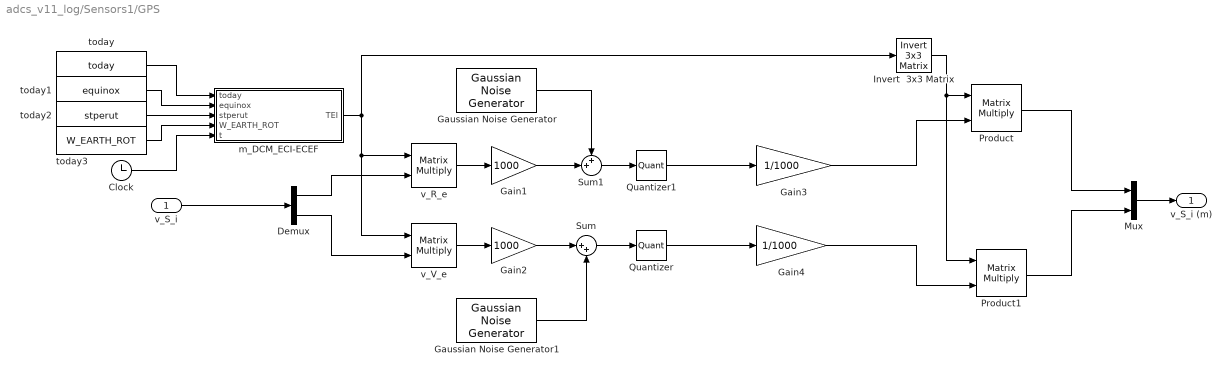
== system adcs_v11_log/Sensors1/GPS ==
  v_S_i : Inport  OutDataType=sfix(16)  OutScaling=2^0
  Clock : Clock
      settings: Decimation=10
  Demux : Demux  Outputs=2
  Gain1 : Gain  Gain=1000  ParameterDataType=sfix(16)  ParameterScaling=2^0  OutDataType=sfix(16)  OutScaling=2^0
  Gain2 : Gain  Gain=1000  ParameterDataType=sfix(16)  ParameterScaling=2^0  OutDataType=sfix(16)  OutScaling=2^0
  Gain3 : Gain  Gain=1/1000  ParameterDataType=sfix(16)  ParameterScaling=2^0  OutDataType=sfix(16)  OutScaling=2^0
  Gain4 : Gain  Gain=1/1000  ParameterDataType=sfix(16)  ParameterScaling=2^0  OutDataType=sfix(16)  OutScaling=2^0
  Gaussian Noise Generator : commnoisgen2/Gaussian Noise Generator  SystemSampleTime=-1  m=0  d=s_x_GPS_X  s=41  Ts=s_SIM_STEP_SIZE  frameBased=off  sampPerFrame=1  orient=off  outDataType=double
  Gaussian Noise Generator1 : commnoisgen2/Gaussian Noise Generator  SystemSampleTime=-1  m=0  d=s_x_GPS_V  s=41  Ts=s_SIM_STEP_SIZE  frameBased=off  sampPerFrame=1  orient=off  outDataType=double
  Invert  3x3 Matrix : aerolibutil/Invert  3x3 Matrix  SystemSampleTime=-1
  Mux : Mux  Inputs=2
  Product : Product  Multiplication=Matrix(*)  OutDataType=sfix(16)  OutScaling=2^0  RndMeth=Zero
  Product1 : Product  Multiplication=Matrix(*)  OutDataType=sfix(16)  OutScaling=2^0  RndMeth=Zero
  Quantizer : Quantizer  QuantizationInterval=1/(2^31)
  Quantizer1 : Quantizer  QuantizationInterval=1/(2^31)
  Sum : Sum  Inputs=|++  OutDataType=sfix(16)  OutScaling=2^0
  Sum1 : Sum  Inputs=++|  OutDataType=sfix(16)  OutScaling=2^0
  m_DCM_ECI-ECEF : Stateflow chart
  today : Constant  Value=today  OutDataType=sfix(16)  OutScaling=2^0
  today1 : Constant  Value=equinox  OutDataType=sfix(16)  OutScaling=2^0
  today2 : Constant  Value=stperut  OutDataType=sfix(16)  OutScaling=2^0
  today3 : Constant  Value=W_EARTH_ROT  OutDataType=sfix(16)  OutScaling=2^0
  v_R_e : Product  Multiplication=Matrix(*)  OutDataType=sfix(16)  OutScaling=2^0  RndMeth=Zero
  v_V_e : Product  Multiplication=Matrix(*)  OutDataType=sfix(16)  OutScaling=2^0  RndMeth=Zero
  v_S_i (m) : Outport  OutDataType=sfix(16)  OutScaling=2^0
  wires:
  Gaussian Noise Generator/1 -> Sum1/1
  Gaussian Noise Generator1/1 -> Sum/2
  Product1/1 -> Mux/2
  Gain4/1 -> Product1/2
  Product/1 -> Mux/1
  Gain3/1 -> Product/2
  Invert  3x3 Matrix/1 -> Product1/1, Product/1
  Quantizer1/1 -> Gain3/1
  Mux/1 -> v_S_i (m)/1
  Sum/1 -> Quantizer/1
  Sum1/1 -> Quantizer1/1
  Gain1/1 -> Sum1/2
  Gain2/1 -> Sum/1
  v_R_e/1 -> Gain1/1
  v_V_e/1 -> Gain2/1
  Quantizer/1 -> Gain4/1
  Clock/1 -> m_DCM_ECI-ECEF/5(t)
  Demux/2 -> v_V_e/2
  Demux/1 -> v_R_e/2
  v_S_i/1 -> Demux/1
  today3/1 -> m_DCM_ECI-ECEF/4(W_EARTH_ROT)
  today2/1 -> m_DCM_ECI-ECEF/3(stperut)
  today1/1 -> m_DCM_ECI-ECEF/2(equinox)
  today/1 -> m_DCM_ECI-ECEF/1(today)
  m_DCM_ECI-ECEF/1(TEI) -> Invert  3x3 Matrix/1, v_V_e/1, v_R_e/1

== system adcs_v11_log/Sensors1/Magnetometer simple ==
  v_B_b : Inport  OutDataType=sfix(16)  OutScaling=2^0
  Constant : Constant  Value=s_x_MAGMETER_BIAS  OutDataType=fixdt(1, 16)  OutScaling=2^0
  Gaussian Noise Generator : commnoisgen2/Gaussian Noise Generator  SystemSampleTime=-1  m=0  d=s_x_MAGMETER  s=41  Ts=s_SIM_STEP_SIZE  frameBased=off  sampPerFrame=1  orient=off  outDataType=double
  Sum1 : Sum  Inputs=+++  OutDataType=sfix(16)  OutScaling=2^0
  v_B_b(m) : Outport  OutDataType=sfix(16)  OutScaling=2^0
  wires:
  Constant/1 -> Sum1/3
  Sum1/1 -> v_B_b(m)/1
  Gaussian Noise Generator/1 -> Sum1/1
  v_B_b/1 -> Sum1/2

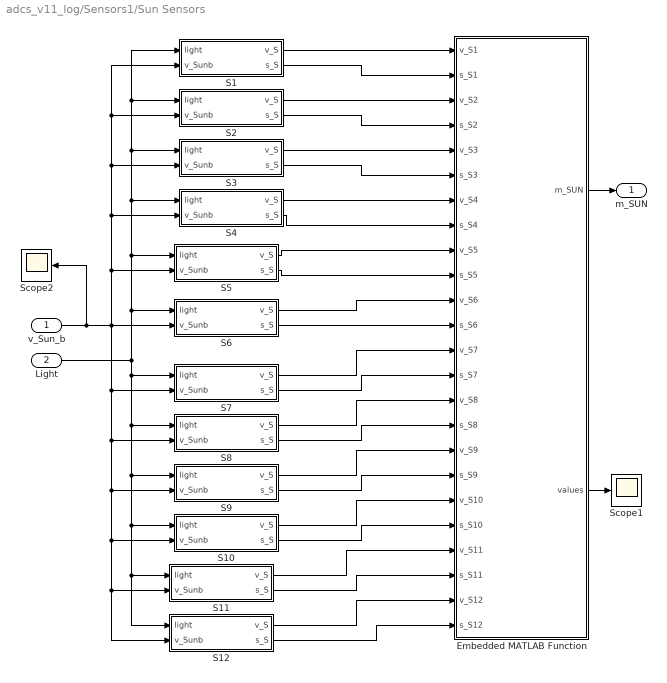
== system adcs_v11_log/Sensors1/Sun Sensors ==
  v_Sun_b : Inport  OutDataType=sfix(16)  OutScaling=2^0
  Light : Inport  Port=2  OutDataType=sfix(16)  OutScaling=2^0
  Embedded MATLAB Function : Stateflow chart
  S1 : Subsystem
  S10 : Subsystem
  S11 : Subsystem
  S12 : Subsystem
  S2 : Subsystem
  S3 : Subsystem
  S4 : Subsystem
  S5 : Subsystem
  S6 : Subsystem
  S7 : Subsystem
  S8 : Subsystem
  S9 : Subsystem
  Scope1 : Scope
      settings: TimeRange=80000  YMin=-6.5  YMax=1  SaveName=ScopeData10  SampleInput=on  SampleTime=5
  Scope2 : Scope
      settings: TimeRange=80000  YMin=-6.5  YMax=1  SaveName=ScopeData12  SampleInput=on  SampleTime=5
  m_SUN : Outport  OutDataType=fixdt(1, 16)  OutScaling=2^0
  wires:
  Light/1 -> S12/1(light), S11/1(light), S10/1(light), S9/1(light), S8/1(light), S7/1(light), S1/1(light), S2/1(light), S3/1(light), S4/1(light), S5/1(light), S6/1(light)
  Embedded MATLAB Function/1(m_SUN) -> m_SUN/1
  v_Sun_b/1 -> S11/2(v_Sunb), S12/2(v_Sunb), S10/2(v_Sunb), S9/2(v_Sunb), S8/2(v_Sunb), S7/2(v_Sunb), S6/2(v_Sunb), S5/2(v_Sunb), S4/2(v_Sunb), S3/2(v_Sunb), S2/2(v_Sunb), S1/2(v_Sunb), Scope2/1
  Embedded MATLAB Function/2(values) -> Scope1/1
  S1/1(v_S) -> Embedded MATLAB Function/1(v_S1)
  S1/2(s_S) -> Embedded MATLAB Function/2(s_S1)
  S2/1(v_S) -> Embedded MATLAB Function/3(v_S2)
  S2/2(s_S) -> Embedded MATLAB Function/4(s_S2)
  S3/1(v_S) -> Embedded MATLAB Function/5(v_S3)
  S3/2(s_S) -> Embedded MATLAB Function/6(s_S3)
  S4/1(v_S) -> Embedded MATLAB Function/7(v_S4)
  S4/2(s_S) -> Embedded MATLAB Function/8(s_S4)
  S5/1(v_S) -> Embedded MATLAB Function/9(v_S5)
  S5/2(s_S) -> Embedded MATLAB Function/10(s_S5)
  S6/1(v_S) -> Embedded MATLAB Function/11(v_S6)
  S6/2(s_S) -> Embedded MATLAB Function/12(s_S6)
  S7/1(v_S) -> Embedded MATLAB Function/13(v_S7)
  S7/2(s_S) -> Embedded MATLAB Function/14(s_S7)
  S8/1(v_S) -> Embedded MATLAB Function/15(v_S8)
  S8/2(s_S) -> Embedded MATLAB Function/16(s_S8)
  S9/1(v_S) -> Embedded MATLAB Function/17(v_S9)
  S9/2(s_S) -> Embedded MATLAB Function/18(s_S9)
  S10/1(v_S) -> Embedded MATLAB Function/19(v_S10)
  S10/2(s_S) -> Embedded MATLAB Function/20(s_S10)
  S11/2(s_S) -> Embedded MATLAB Function/22(s_S11)
  S12/1(v_S) -> Embedded MATLAB Function/23(v_S12)
  S12/2(s_S) -> Embedded MATLAB Function/24(s_S12)
  S11/1(v_S) -> Embedded MATLAB Function/21(v_S11)

== system adcs_v11_log/WMM/state vector to v_Bi ==
  v_S_i : Inport  OutDataType=sfix(16)  OutScaling=2^0
  Demux : Demux  Outputs=2
  Invert  3x3 Matrix : aerolibutil/Invert  3x3 Matrix  SystemSampleTime=-1
  Magnetic field v_Be : Subsystem
  Subsystem : Subsystem
  Terminator : Terminator
  v_Bi : Product  Multiplication=Matrix(*)  OutDataType=sfix(16)  OutScaling=2^0  RndMeth=Zero
  v_Vi1 : Product  Multiplication=Matrix(*)  OutDataType=sfix(16)  OutScaling=2^0  RndMeth=Zero
  v_B_I : Outport  OutDataType=sfix(16)  OutScaling=2^0
  wires:
  v_Bi/1 -> v_B_I/1
  Demux/1 -> v_Vi1/2
  v_S_i/1 -> Demux/1
  Demux/2 -> Terminator/1
  v_Vi1/1 -> Magnetic field v_Be/1(XYZ-ECEF)
  Subsystem/1(TEI) -> v_Vi1/1, Invert  3x3 Matrix/1
  Magnetic field v_Be/1("v_B_e (T) ") -> v_Bi/2
  Invert  3x3 Matrix/1 -> v_Bi/1

== system adcs_v11_log/q -> w/LPF ==
  "w " : Inport
  Demux1 : Demux  Outputs=3
  Discrete 1st-Order Filter : powerlib_extras/Discrete  Control Blocks/Discrete 1st-Order Filter  DialogController=POWERSYS.PowerSysDialog  SystemSampleTime=-1  FilterType=Lowpass  Tc=s_TAU_W  Ts=s_FRAME_SIZE  Initialize=off  Vac_Init=[0.8 -25 60]  Vdc_Init=-0.4  PlotResponse=off  param1=[1 500 0.1]
  Discrete 1st-Order Filter1 : powerlib_extras/Discrete  Control Blocks/Discrete 1st-Order Filter  DialogController=POWERSYS.PowerSysDialog  SystemSampleTime=-1  FilterType=Lowpass  Tc=s_TAU_W  Ts=s_FRAME_SIZE  Initialize=off  Vac_Init=[0.8 -25 60]  Vdc_Init=-0.4  PlotResponse=off  param1=[1 500 0.1]
  Discrete 1st-Order Filter2 : powerlib_extras/Discrete  Control Blocks/Discrete 1st-Order Filter  DialogController=POWERSYS.PowerSysDialog  SystemSampleTime=-1  FilterType=Lowpass  Tc=s_TAU_W  Ts=s_FRAME_SIZE  Initialize=off  Vac_Init=[0.8 -25 60]  Vdc_Init=-0.4  PlotResponse=off  param1=[1 500 0.1]
  Mux : Mux  Inputs=3
  w_LPF : Outport
  wires:
  Mux/1 -> w_LPF/1
  "w "/1 -> Demux1/1
  Discrete 1st-Order Filter2/1 -> Mux/3
  Discrete 1st-Order Filter/1 -> Mux/1
  Discrete 1st-Order Filter1/1 -> Mux/2
  Demux1/3 -> Discrete 1st-Order Filter2/1
  Demux1/2 -> Discrete 1st-Order Filter1/1
  Demux1/1 -> Discrete 1st-Order Filter/1

== system adcs_v11_log/q -> w/Subsystem4 ==
  \ : Inport
  Constant : Constant  Value=s_FRAME_SIZE  OutDataType=fixdt(1, 16)  OutScaling=2^0
  Variable Time Delay : VariableTransportDelay  MaximumDelay=10000
  =>\ : Outport
  wires:
  Constant/1 -> Variable Time Delay/2
  \/1 -> Variable Time Delay/1
  Variable Time Delay/1 -> =>\/1

== system adcs_v11_log/q -> w/Subsystem6 ==
  light : Inport  OutDataType=fixdt(1, 16)  OutScaling=2^0
  Embedded MATLAB Function : Stateflow chart
  Embedded MATLAB Function1 : Stateflow chart
  Integer Delay : simulink/Discrete/Integer Delay  vinit=0.0  samptime=-1  NumDelays=3000
  Scope : Scope
  Scope1 : Scope
  Scope2 : Scope
      settings: SaveName=ScopeData2
  w-ctrl : Outport  OutDataType=fixdt(1, 16)  OutScaling=2^0
  wires:
  Embedded MATLAB Function1/1(y) -> Embedded MATLAB Function/1(a)
  Integer Delay/1 -> Embedded MATLAB Function/2(b), Scope1/1
  light/1 -> Scope2/1, Integer Delay/1, Embedded MATLAB Function1/1(u)
  Embedded MATLAB Function/1(y) -> Scope/1, w-ctrl/1

== system adcs_v11_log/External Torques/Aerodynamic  Torque/Subsystem ==
  Clock : Clock
      settings: Decimation=10
  m_DCM_ECI-ECEF2 : Stateflow chart
  today : Constant  Value=today  OutDataType=sfix(16)  OutScaling=2^0
  today1 : Constant  Value=equinox  OutDataType=sfix(16)  OutScaling=2^0
  today2 : Constant  Value=stperut  OutDataType=sfix(16)  OutScaling=2^0
  today3 : Constant  Value=W_EARTH_ROT  OutDataType=sfix(16)  OutScaling=2^0
  TEI : Outport
  wires:
  today/1 -> m_DCM_ECI-ECEF2/1(today)
  today1/1 -> m_DCM_ECI-ECEF2/2(equinox)
  today2/1 -> m_DCM_ECI-ECEF2/3(stperut)
  today3/1 -> m_DCM_ECI-ECEF2/4(W_EARTH_ROT)
  Clock/1 -> m_DCM_ECI-ECEF2/5(t)
  m_DCM_ECI-ECEF2/1(TEI) -> TEI/1

== system adcs_v11_log/Satellite Computations I Propagators/Orbit propagator model/Subsystem1 ==
  v : Inport
  Pulse Generator : DiscretePulseGenerator  PulseType=Time based  Amplitude=1  Period=s_FRAME_SIZE  PulseWidth=50  PhaseDelay=0  SampleTime=1
  Sample and Hold : dspsigops/Sample and Hold  SystemSampleTime=-1  trig=Rising edge  initCond=v_Si0(4:6)  latchinput=off
  v(H) : Outport
  wires:
  Sample and Hold/1 -> v(H)/1
  v/1 -> Sample and Hold/1
  Pulse Generator/1 -> Sample and Hold/Trigger

== system adcs_v11_log/Satellite Computations I Propagators/Orbit propagator model/Subsystem3 ==
  v : Inport
  Pulse Generator : DiscretePulseGenerator  PulseType=Time based  Amplitude=1  Period=s_FRAME_SIZE  PulseWidth=50  PhaseDelay=0  SampleTime=1
  Sample and Hold : dspsigops/Sample and Hold  SystemSampleTime=-1  trig=Rising edge  initCond=v_Si0(1:3)  latchinput=off
  v(H) : Outport
  wires:
  Pulse Generator/1 -> Sample and Hold/Trigger
  v/1 -> Sample and Hold/1
  Sample and Hold/1 -> v(H)/1

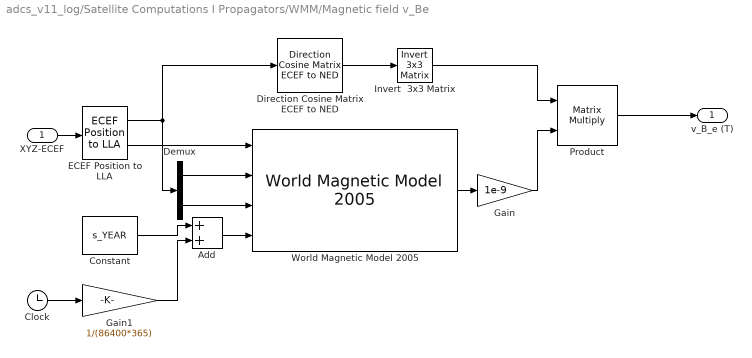
== system adcs_v11_log/Satellite Computations I Propagators/WMM/Magnetic field v_Be ==
  XYZ-ECEF : Inport  OutDataType=sfix(16)  OutScaling=2^0
  Add : Sum  OutDataType=sfix(16)  OutScaling=2^-10
  Clock : Clock
      settings: Decimation=10
  Constant : Constant  Value=s_YEAR  OutDataType=sfix(16)  OutScaling=2^0
  Demux : Demux  Outputs=2
  Direction Cosine Matrix ECEF to NED : aerolibtransform2/Direction Cosine Matrix ECEF to NED  SystemSampleTime=-1
  ECEF Position to LLA : aerolibtransform2/ECEF Position to LLA  SystemSampleTime=-1  units=Metric (MKS)  ptype=Earth (WGS84)  F=1/298.257223563  R=6378137
  Gain : Gain  Gain=1e-9  ParameterDataType=sfix(16)  ParameterScaling=2^0  OutDataType=sfix(16)  OutScaling=2^0
  Gain1 : Gain  Gain=1/(86400*365)  ParameterDataType=sfix(16)  ParameterScaling=2^0  OutDataType=sfix(16)  OutScaling=2^0
  Invert  3x3 Matrix : aerolibutil/Invert  3x3 Matrix  SystemSampleTime=-1
  Product : Product  Multiplication=Matrix(*)  OutDataType=sfix(16)  OutScaling=2^0  RndMeth=Zero
  World Magnetic Model 2005 : aerolibgravity2/World Magnetic Model 2005  SystemSampleTime=-1  units=Metric (MKS)  time_in=on  month=January  day=1  year=2005  action=None  h_out=off  dec_out=off  inc_out=off  ti_out=off
  "v_B_e (T) " : Outport  OutDataType=sfix(16)  OutScaling=2^0
  wires:
  Gain1/1 -> Add/2
  Clock/1 -> Gain1/1
  Add/1 -> World Magnetic Model 2005/4
  Constant/1 -> Add/1
  XYZ-ECEF/1 -> ECEF Position to LLA/1
  ECEF Position to LLA/1 -> Demux/1, Direction Cosine Matrix ECEF to NED/1
  ECEF Position to LLA/2 -> World Magnetic Model 2005/1
  Demux/1 -> World Magnetic Model 2005/2
  Demux/2 -> World Magnetic Model 2005/3
  Direction Cosine Matrix ECEF to NED/1 -> Invert  3x3 Matrix/1
  Invert  3x3 Matrix/1 -> Product/1
  Product/1 -> "v_B_e (T) "/1
  World Magnetic Model 2005/1 -> Gain/1
  Gain/1 -> Product/2

== system adcs_v11_log/Satellite Computations I Propagators/WMM/Subsystem ==
  Clock : Clock
      settings: Decimation=10
  m_DCM_ECI-ECEF2 : Stateflow chart
  today : Constant  Value=today  OutDataType=sfix(16)  OutScaling=2^0
  today1 : Constant  Value=equinox  OutDataType=sfix(16)  OutScaling=2^0
  today2 : Constant  Value=stperut  OutDataType=sfix(16)  OutScaling=2^0
  today3 : Constant  Value=W_EARTH_ROT  OutDataType=sfix(16)  OutScaling=2^0
  TEI : Outport
  wires:
  m_DCM_ECI-ECEF2/1(TEI) -> TEI/1
  Clock/1 -> m_DCM_ECI-ECEF2/5(t)
  today3/1 -> m_DCM_ECI-ECEF2/4(W_EARTH_ROT)
  today2/1 -> m_DCM_ECI-ECEF2/3(stperut)
  today1/1 -> m_DCM_ECI-ECEF2/2(equinox)
  today/1 -> m_DCM_ECI-ECEF2/1(today)
